simulink model "HevP2ReferenceApplication"  (R2023a)
settings: Solver=ode23tb  StartTime=0  StopTime=1000  RelTol=1e-2  EnableMultiTasking=on
undefined symbols (not defined in the file): at, SOCLast, Stuck
libraries: simulink x5, SignalEditorBlockLib x4, autolibshared x2, FIBlockLib x2
(part 2 of 2)

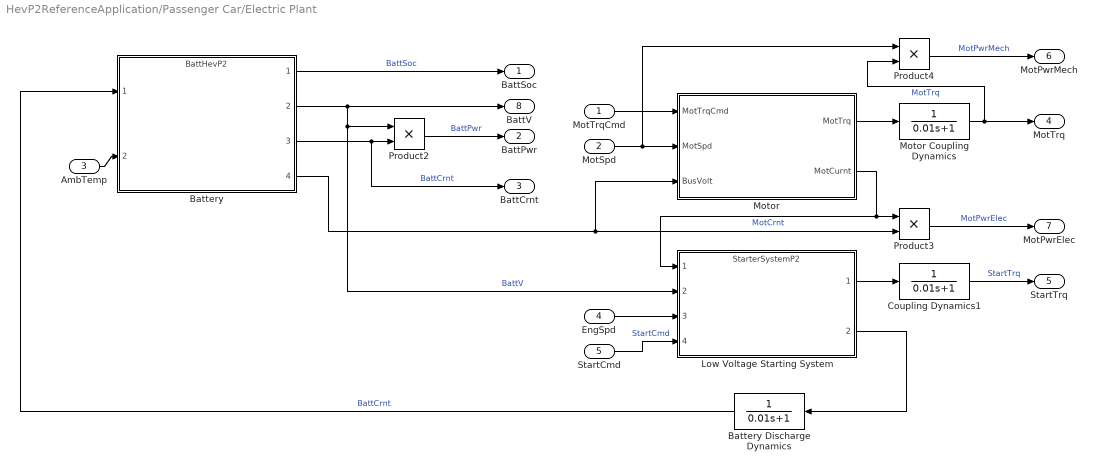
== system HevP2ReferenceApplication/Passenger Car/Electric Plant ==
  MotTrqCmd : Inport
  MotSpd : Inport  Port=2
  AmbTemp : Inport  Port=3
  EngSpd : Inport  Port=4
  StartCmd : Inport  Port=5
  Battery : ModelReference  ModelNameDialog=BattHevP2.slx  SimulationMode=Normal  ModelReferenceVersion=7.0
  Battery Discharge Dynamics : TransferFcn  Denominator=[0.01 1]
  Coupling Dynamics1 : TransferFcn  Denominator=[0.01 1]
  Low Voltage Starting System : ModelReference  ModelNameDialog=StarterSystemP2.slx  SimulationMode=Normal  ModelReferenceVersion=9.1
  Motor : Subsystem  Variant=on  VariantControlMode=label  LabelModeActiveChoice=MotMapped
  Motor Coupling Dynamics : TransferFcn  Denominator=[0.01 1]
  Product2 : Product
  Product3 : Product
  Product4 : Product
  BattSoc : Outport  VectorParamsAs1DForOutWhenUnconnected=off
  BattPwr : Outport  Port=2  VectorParamsAs1DForOutWhenUnconnected=off
  BattCrnt : Outport  Port=3  VectorParamsAs1DForOutWhenUnconnected=off
  MotTrq : Outport  Port=4  VectorParamsAs1DForOutWhenUnconnected=off
  StartTrq : Outport  Port=5  VectorParamsAs1DForOutWhenUnconnected=off
  MotPwrMech : Outport  Port=6  VectorParamsAs1DForOutWhenUnconnected=off
  MotPwrElec : Outport  Port=7  VectorParamsAs1DForOutWhenUnconnected=off
  BattV : Outport  Port=8  VectorParamsAs1DForOutWhenUnconnected=off
  wires:
  Battery/2 -> Low Voltage Starting System/2, Product2/1, BattV/1  "BattV"
  Battery/1 -> BattSoc/1  "BattSoc"
  MotSpd/1 -> Product4/1, Motor/2(MotSpd)
  MotTrqCmd/1 -> Motor/1(MotTrqCmd)
  AmbTemp/1 -> Battery/2
  Product2/1 -> BattPwr/1  "BattPwr"
  Motor/1(MotTrq) -> Motor Coupling Dynamics/1
  Motor Coupling Dynamics/1 -> Product4/2, MotTrq/1  "MotTrq"
  Low Voltage Starting System/2 -> Battery Discharge Dynamics/1
  Motor/2(MotCurnt) -> Low Voltage Starting System/1, Product3/1  "MotCrnt"
  EngSpd/1 -> Low Voltage Starting System/3
  StartCmd/1 -> Low Voltage Starting System/4  "StartCmd"
  Low Voltage Starting System/1 -> Coupling Dynamics1/1
  Product4/1 -> MotPwrMech/1  "MotPwrMech"
  Product3/1 -> MotPwrElec/1  "MotPwrElec"
  Battery Discharge Dynamics/1 -> Battery/1  "BattCrnt"
  Coupling Dynamics1/1 -> StartTrq/1  "StartTrq"
  Battery/3 -> Product2/2, BattCrnt/1  "BattCrnt"
  Battery/4 -> Motor/3(BusVolt), Product3/2

== system HevP2ReferenceApplication/Passenger Car/Electric Plant Input ==
  Ctrl : Inport
  Veh : Inport  Port=2
  Env : Inport  Port=3
  EngFdbk : Inport  Port=4
  Bus Selector : BusSelector  OutputSignals=PtCtrl.MotTrqCmd,PtCtrl.StartCmd
  Bus Selector1 : BusSelector  OutputSignals=MotSpd
  Bus Selector2 : BusSelector  OutputSignals=Temp
  Bus Selector3 : BusSelector  OutputSignals=EngSpd
  First Order Hold : FirstOrderHold  OutputAlgorithm=Fast (Minimize Error)  ErrorTolerance=10e6
  First Order Hold1 : FirstOrderHold  ErrorTolerance=10e6
  MotTrqCmd : Outport  VectorParamsAs1DForOutWhenUnconnected=off
  MotSpd : Outport  Port=2  VectorParamsAs1DForOutWhenUnconnected=off
  AmbTemp : Outport  Port=3  VectorParamsAs1DForOutWhenUnconnected=off
  EngSpd : Outport  Port=4  VectorParamsAs1DForOutWhenUnconnected=off
  StartCmd : Outport  Port=5  VectorParamsAs1DForOutWhenUnconnected=off
  wires:
  First Order Hold1/1 -> StartCmd/1  "StartCmd"
  Bus Selector3/1 -> EngSpd/1  "<EngSpd>"
  EngFdbk/1 -> Bus Selector3/1
  Bus Selector2/1 -> AmbTemp/1  "<Temp>"
  Env/1 -> Bus Selector2/1
  Bus Selector1/1 -> MotSpd/1  "<MotSpd>"
  Veh/1 -> Bus Selector1/1
  Bus Selector/1 -> First Order Hold/1  "<MotTrqCmd>"
  Ctrl/1 -> Bus Selector/1
  First Order Hold/1 -> MotTrqCmd/1  "MotTrqCmd"
  Bus Selector/2 -> First Order Hold1/1  "<StartCmd>"

== system HevP2ReferenceApplication/Passenger Car/Electric Plant Output ==
  BattSoc : Inport
  BattPwr : Inport  Port=2
  BattCrnt : Inport  Port=3
  MotTrq : Inport  Port=4
  StartTrq : Inport  Port=5
  MotPwrMech : Inport  Port=6
  MotPwrElec : Inport  Port=7
  BattV : Inport  Port=8
  Bus Creator1 : BusCreator  Inputs=8
  ElecFdbk : Outport  VectorParamsAs1DForOutWhenUnconnected=off
  wires:
  BattV/1 -> Bus Creator1/8
  MotPwrElec/1 -> Bus Creator1/7
  MotPwrMech/1 -> Bus Creator1/6
  StartTrq/1 -> Bus Creator1/5
  MotTrq/1 -> Bus Creator1/4
  BattCrnt/1 -> Bus Creator1/3
  BattSoc/1 -> Bus Creator1/1
  BattPwr/1 -> Bus Creator1/2
  Bus Creator1/1 -> ElecFdbk/1  "ElecFdbk"

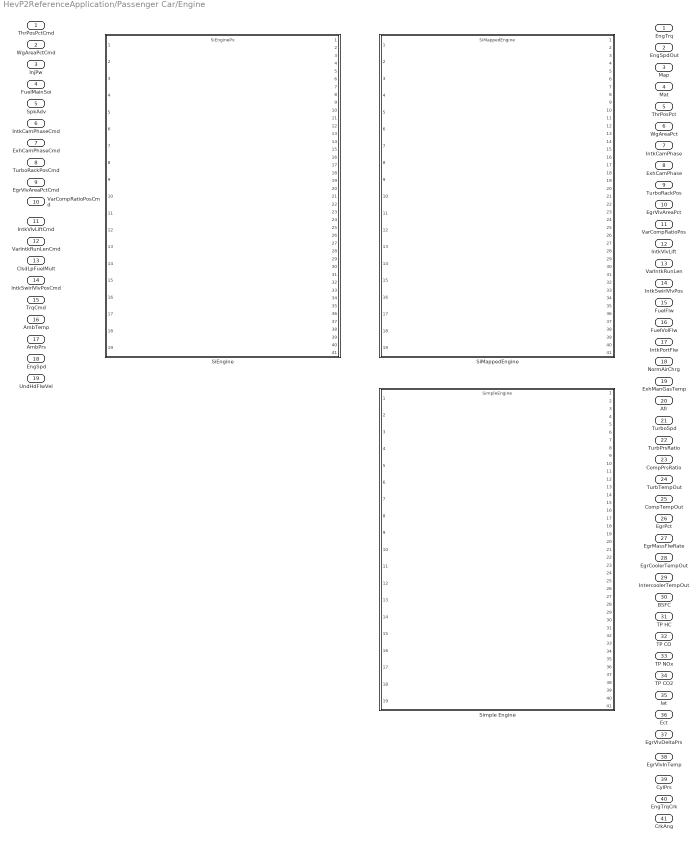
== system HevP2ReferenceApplication/Passenger Car/Engine ==
  ThrPosPctCmd : Inport
  WgAreaPctCmd : Inport  Port=2
  InjPw : Inport  Port=3
  FuelMainSoi : Inport  Port=4
  SpkAdv : Inport  Port=5
  IntkCamPhaseCmd : Inport  Port=6
  ExhCamPhaseCmd : Inport  Port=7
  TurboRackPosCmd : Inport  Port=8
  EgrVlvAreaPctCmd : Inport  Port=9
  VarCompRatioPosCmd : Inport  Port=10
  IntkVlvLiftCmd : Inport  Port=11
  VarIntkRunLenCmd : Inport  Port=12
  ClsdLpFuelMult : Inport  Port=13
  IntkSwirlVlvPosCmd : Inport  Port=14
  TrqCmd : Inport  Port=15
  AmbTemp : Inport  Port=16
  AmbPrs : Inport  Port=17
  EngSpd : Inport  Port=18
  UndHdFlwVel : Inport  Port=19
  SiEngine : ModelReference  ModelNameDialog=SiEnginePx.slx  SimulationMode=Normal  VariantControl=SiEngine  ModelReferenceVersion=6.0
  SiMappedEngine : ModelReference  ModelNameDialog=SiMappedEngine.slx  SimulationMode=Normal  VariantControl=SiMappedEngine  ModelReferenceVersion=6.0
  Simple Engine : ModelReference  ModelNameDialog=SimpleEngine.slx  SimulationMode=Normal  VariantControl=Simple Engine  ModelReferenceVersion=6.0
  EngTrq : Outport  VectorParamsAs1DForOutWhenUnconnected=off
  EngSpdOut : Outport  Port=2  VectorParamsAs1DForOutWhenUnconnected=off
  Map : Outport  Port=3  VectorParamsAs1DForOutWhenUnconnected=off
  Mat : Outport  Port=4  VectorParamsAs1DForOutWhenUnconnected=off
  ThrPosPct : Outport  Port=5  VectorParamsAs1DForOutWhenUnconnected=off
  WgAreaPct : Outport  Port=6  VectorParamsAs1DForOutWhenUnconnected=off
  IntkCamPhase : Outport  Port=7  VectorParamsAs1DForOutWhenUnconnected=off
  ExhCamPhase : Outport  Port=8  VectorParamsAs1DForOutWhenUnconnected=off
  TurboRackPos : Outport  Port=9  VectorParamsAs1DForOutWhenUnconnected=off
  EgrVlvAreaPct : Outport  Port=10  VectorParamsAs1DForOutWhenUnconnected=off
  VarCompRatioPos : Outport  Port=11  VectorParamsAs1DForOutWhenUnconnected=off
  IntkVlvLift : Outport  Port=12  VectorParamsAs1DForOutWhenUnconnected=off
  VarIntkRunLen : Outport  Port=13  VectorParamsAs1DForOutWhenUnconnected=off
  IntkSwirlVlvPos : Outport  Port=14  VectorParamsAs1DForOutWhenUnconnected=off
  FuelFlw : Outport  Port=15  VectorParamsAs1DForOutWhenUnconnected=off
  FuelVolFlw : Outport  Port=16  VectorParamsAs1DForOutWhenUnconnected=off
  IntkPortFlw : Outport  Port=17  VectorParamsAs1DForOutWhenUnconnected=off
  NormAirChrg : Outport  Port=18  VectorParamsAs1DForOutWhenUnconnected=off
  ExhManGasTemp : Outport  Port=19  VectorParamsAs1DForOutWhenUnconnected=off
  Afr : Outport  Port=20  VectorParamsAs1DForOutWhenUnconnected=off
  TurboSpd : Outport  Port=21  VectorParamsAs1DForOutWhenUnconnected=off
  TurbPrsRatio : Outport  Port=22  VectorParamsAs1DForOutWhenUnconnected=off
  CompPrsRatio : Outport  Port=23  VectorParamsAs1DForOutWhenUnconnected=off
  TurbTempOut : Outport  Port=24  VectorParamsAs1DForOutWhenUnconnected=off
  CompTempOut : Outport  Port=25  VectorParamsAs1DForOutWhenUnconnected=off
  EgrPct : Outport  Port=26  VectorParamsAs1DForOutWhenUnconnected=off
  EgrMassFlwRate : Outport  Port=27  VectorParamsAs1DForOutWhenUnconnected=off
  EgrCoolerTempOut : Outport  Port=28  VectorParamsAs1DForOutWhenUnconnected=off
  IntercoolerTempOut : Outport  Port=29  VectorParamsAs1DForOutWhenUnconnected=off
  BSFC : Outport  Port=30  VectorParamsAs1DForOutWhenUnconnected=off
  TP HC : Outport  Port=31  VectorParamsAs1DForOutWhenUnconnected=off
  TP CO : Outport  Port=32  VectorParamsAs1DForOutWhenUnconnected=off
  TP NOx : Outport  Port=33  VectorParamsAs1DForOutWhenUnconnected=off
  TP CO2 : Outport  Port=34  VectorParamsAs1DForOutWhenUnconnected=off
  Iat : Outport  Port=35  VectorParamsAs1DForOutWhenUnconnected=off
  Ect : Outport  Port=36  VectorParamsAs1DForOutWhenUnconnected=off
  EgrVlvDeltaPrs : Outport  Port=37  VectorParamsAs1DForOutWhenUnconnected=off
  EgrVlvInTemp : Outport  Port=38  VectorParamsAs1DForOutWhenUnconnected=off
  CylPrs : Outport  Port=39  VectorParamsAs1DForOutWhenUnconnected=off
  EngTrqCrk : Outport  Port=40  VectorParamsAs1DForOutWhenUnconnected=off
  CrkAng : Outport  Port=41  VectorParamsAs1DForOutWhenUnconnected=off

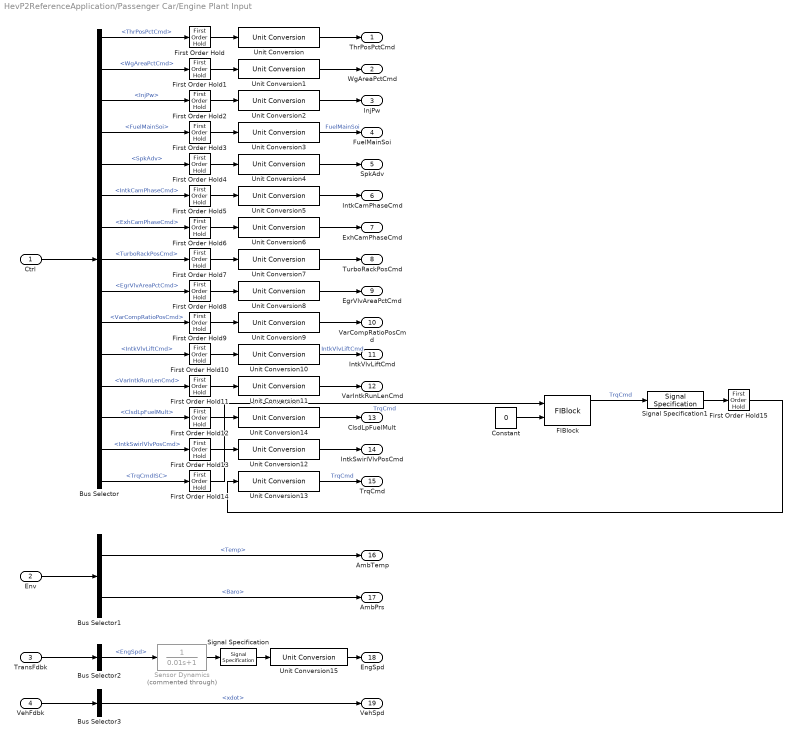
== system HevP2ReferenceApplication/Passenger Car/Engine Plant Input ==
  Ctrl : Inport
  Env : Inport  Port=2
  TransFdbk : Inport  Port=3
  VehFdbk : Inport  Port=4
  Bus Selector : BusSelector  OutputSignals=EngCtrl.ThrPosPctCmd,EngCtrl.WgAreaPctCmd,EngCtrl.InjPw,EngCtrl.FuelMainSoi,EngCtrl.SpkAdv,EngCtrl.IntkCamPhaseCmd,EngCtrl.ExhCamPhaseCmd,EngCtrl.TurboRackPosCmd,EngCtrl.EgrVlvAreaPctCmd,EngCtrl.VarCompRatioPosCmd,EngCtrl.IntkVlvLiftCmd,EngCtrl.VarIntkRunLenCmd,EngCtrl.ClsdLpFuelMult,EngCtrl.IntkSwirlVlvPosCmd,EngCtrl.TrqCmdISC
  Bus Selector1 : BusSelector  OutputSignals=Temp,Baro
  Bus Selector2 : BusSelector  OutputSignals=EngSpd
  Bus Selector3 : BusSelector  OutputSignals=xdot
  Constant : Constant  Value=0
  FIBlock : FIBlockLib/FIBlock  FIBlockName=2  FInjEnable=off  FaultType=Stuck-at  FaultValue=1  FaultEvent=Deterministic  EventValue=50  FaultEffect=Infinite time  EffectValue=0
      settings: SourceProductName=Fault Injection block
  First Order Hold : FirstOrderHold  ErrorTolerance=10e6
  First Order Hold1 : FirstOrderHold  ErrorTolerance=10e6
  First Order Hold{3..14} (12 alike) : FirstOrderHold  ErrorTolerance=10e6  AllowContinuousInput=on
  First Order Hold15 : FirstOrderHold  ErrorTolerance=inf
  First Order Hold2 : FirstOrderHold  ErrorTolerance=10e6
  Sensor Dynamics : TransferFcn  Commented=through  Denominator=[0.01 1]
  Signal Specification : SignalSpecification  Unit=rad/s
  Signal Specification1 : SignalSpecification  Unit=N*m
  Unit Conversion{,1..12,14..15} (15 alike) : UnitConversion
  Unit Conversion13 : UnitConversion  OutputType=Inherit: Inherit via back propagation
  ThrPosPctCmd : Outport  VectorParamsAs1DForOutWhenUnconnected=off
  WgAreaPctCmd : Outport  Port=2  VectorParamsAs1DForOutWhenUnconnected=off
  InjPw : Outport  Port=3  VectorParamsAs1DForOutWhenUnconnected=off
  FuelMainSoi : Outport  Port=4  VectorParamsAs1DForOutWhenUnconnected=off
  SpkAdv : Outport  Port=5  VectorParamsAs1DForOutWhenUnconnected=off
  IntkCamPhaseCmd : Outport  Port=6  VectorParamsAs1DForOutWhenUnconnected=off
  ExhCamPhaseCmd : Outport  Port=7  VectorParamsAs1DForOutWhenUnconnected=off
  TurboRackPosCmd : Outport  Port=8  VectorParamsAs1DForOutWhenUnconnected=off
  EgrVlvAreaPctCmd : Outport  Port=9  VectorParamsAs1DForOutWhenUnconnected=off
  VarCompRatioPosCmd : Outport  Port=10  VectorParamsAs1DForOutWhenUnconnected=off
  IntkVlvLiftCmd : Outport  Port=11  VectorParamsAs1DForOutWhenUnconnected=off
  VarIntkRunLenCmd : Outport  Port=12  VectorParamsAs1DForOutWhenUnconnected=off
  ClsdLpFuelMult : Outport  Port=13  VectorParamsAs1DForOutWhenUnconnected=off
  IntkSwirlVlvPosCmd : Outport  Port=14  VectorParamsAs1DForOutWhenUnconnected=off
  TrqCmd : Outport  Port=15  VectorParamsAs1DForOutWhenUnconnected=off
  AmbTemp : Outport  Port=16  VectorParamsAs1DForOutWhenUnconnected=off
  AmbPrs : Outport  Port=17  VectorParamsAs1DForOutWhenUnconnected=off
  EngSpd : Outport  Port=18  VectorParamsAs1DForOutWhenUnconnected=off
  VehSpd : Outport  Port=19  VectorParamsAs1DForOutWhenUnconnected=off
  wires:
  Env/1 -> Bus Selector1/1
  Bus Selector1/2 -> AmbPrs/1  "<Baro>"
  TransFdbk/1 -> Bus Selector2/1
  Bus Selector2/1 -> Sensor Dynamics/1  "<EngSpd>"
  Bus Selector1/1 -> AmbTemp/1  "<Temp>"
  VehFdbk/1 -> Bus Selector3/1
  Bus Selector3/1 -> VehSpd/1  "<xdot>"
  Sensor Dynamics/1 -> Signal Specification/1
  Ctrl/1 -> Bus Selector/1
  First Order Hold13/1 -> Unit Conversion12/1
  First Order Hold12/1 -> Unit Conversion14/1
  First Order Hold11/1 -> Unit Conversion11/1
  First Order Hold10/1 -> Unit Conversion10/1
  First Order Hold9/1 -> Unit Conversion9/1
  First Order Hold3/1 -> Unit Conversion3/1
  First Order Hold/1 -> Unit Conversion/1
  First Order Hold1/1 -> Unit Conversion1/1
  First Order Hold2/1 -> Unit Conversion2/1
  First Order Hold4/1 -> Unit Conversion4/1
  First Order Hold5/1 -> Unit Conversion5/1
  First Order Hold6/1 -> Unit Conversion6/1
  First Order Hold7/1 -> Unit Conversion7/1
  First Order Hold8/1 -> Unit Conversion8/1
  Bus Selector/1 -> First Order Hold/1  "<ThrPosPctCmd>"
  Bus Selector/2 -> First Order Hold1/1  "<WgAreaPctCmd>"
  Bus Selector/3 -> First Order Hold2/1  "<InjPw>"
  Bus Selector/4 -> First Order Hold3/1  "<FuelMainSoi>"
  Bus Selector/5 -> First Order Hold4/1  "<SpkAdv>"
  Bus Selector/6 -> First Order Hold5/1  "<IntkCamPhaseCmd>"
  Bus Selector/7 -> First Order Hold6/1  "<ExhCamPhaseCmd>"
  Bus Selector/8 -> First Order Hold7/1  "<TurboRackPosCmd>"
  Bus Selector/9 -> First Order Hold8/1  "<EgrVlvAreaPctCmd>"
  Bus Selector/10 -> First Order Hold9/1  "<VarCompRatioPosCmd>"
  Bus Selector/11 -> First Order Hold10/1  "<IntkVlvLiftCmd>"
  Bus Selector/12 -> First Order Hold11/1  "<VarIntkRunLenCmd>"
  Bus Selector/13 -> First Order Hold12/1  "<ClsdLpFuelMult>"
  Bus Selector/14 -> First Order Hold13/1  "<IntkSwirlVlvPosCmd>"
  Bus Selector/15 -> First Order Hold14/1  "<TrqCmdISC>"
  Unit Conversion11/1 -> VarIntkRunLenCmd/1
  Unit Conversion8/1 -> EgrVlvAreaPctCmd/1
  Unit Conversion12/1 -> IntkSwirlVlvPosCmd/1
  Unit Conversion14/1 -> ClsdLpFuelMult/1
  Unit Conversion/1 -> ThrPosPctCmd/1
  Unit Conversion1/1 -> WgAreaPctCmd/1
  Unit Conversion3/1 -> FuelMainSoi/1  "FuelMainSoi"
  Unit Conversion2/1 -> InjPw/1
  Unit Conversion9/1 -> VarCompRatioPosCmd/1
  Unit Conversion4/1 -> SpkAdv/1
  Unit Conversion7/1 -> TurboRackPosCmd/1
  Unit Conversion13/1 -> TrqCmd/1  "TrqCmd"
  Unit Conversion10/1 -> IntkVlvLiftCmd/1  "IntkVlvLiftCmd"
  Unit Conversion6/1 -> ExhCamPhaseCmd/1
  Unit Conversion5/1 -> IntkCamPhaseCmd/1
  Unit Conversion15/1 -> EngSpd/1
  Signal Specification/1 -> Unit Conversion15/1
  First Order Hold14/1 -> FIBlock/1  "TrqCmd"
  FIBlock/1 -> Signal Specification1/1  "TrqCmd"
  Constant/1 -> FIBlock/2
  Signal Specification1/1 -> First Order Hold15/1
  First Order Hold15/1 -> Unit Conversion13/1

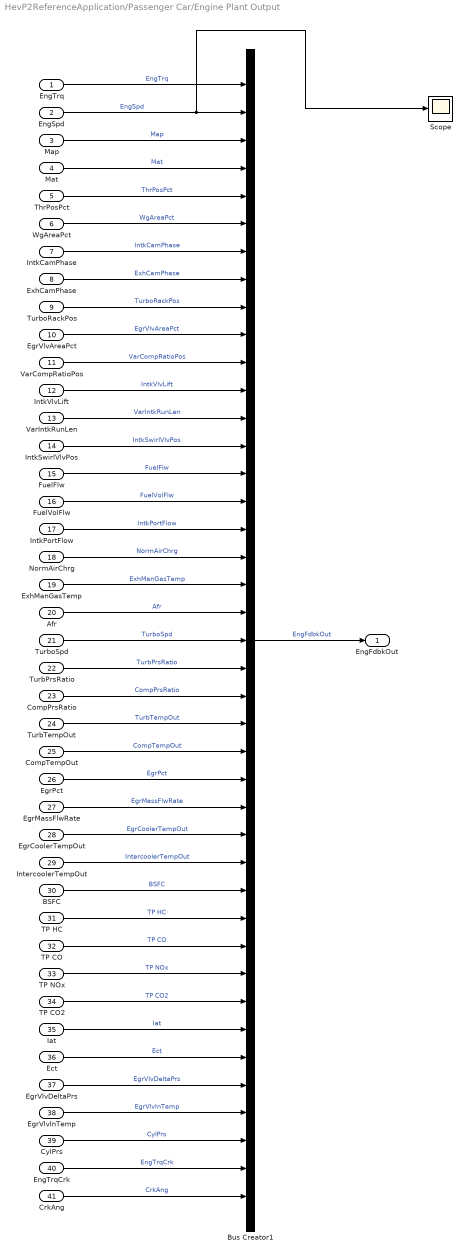
== system HevP2ReferenceApplication/Passenger Car/Engine Plant Output ==
  EngTrq : Inport
  EngSpd : Inport  Port=2
  Map : Inport  Port=3
  Mat : Inport  Port=4
  ThrPosPct : Inport  Port=5
  WgAreaPct : Inport  Port=6
  IntkCamPhase : Inport  Port=7
  ExhCamPhase : Inport  Port=8
  TurboRackPos : Inport  Port=9
  EgrVlvAreaPct : Inport  Port=10
  VarCompRatioPos : Inport  Port=11
  IntkVlvLift : Inport  Port=12
  VarIntkRunLen : Inport  Port=13
  IntkSwirlVlvPos : Inport  Port=14
  FuelFlw : Inport  Port=15
  FuelVolFlw : Inport  Port=16
  IntkPortFlow : Inport  Port=17
  NormAirChrg : Inport  Port=18
  ExhManGasTemp : Inport  Port=19
  Afr : Inport  Port=20
  TurboSpd : Inport  Port=21
  TurbPrsRatio : Inport  Port=22
  CompPrsRatio : Inport  Port=23
  TurbTempOut : Inport  Port=24
  CompTempOut : Inport  Port=25
  EgrPct : Inport  Port=26
  EgrMassFlwRate : Inport  Port=27
  EgrCoolerTempOut : Inport  Port=28
  IntercoolerTempOut : Inport  Port=29
  BSFC : Inport  Port=30
  TP HC : Inport  Port=31
  TP CO : Inport  Port=32
  TP NOx : Inport  Port=33
  TP CO2 : Inport  Port=34
  Iat : Inport  Port=35
  Ect : Inport  Port=36
  EgrVlvDeltaPrs : Inport  Port=37
  EgrVlvInTemp : Inport  Port=38
  CylPrs : Inport  Port=39
  EngTrqCrk : Inport  Port=40
  CrkAng : Inport  Port=41
  Bus Creator1 : BusCreator  Inputs=41
  Scope : Scope
  EngFdbkOut : Outport  VectorParamsAs1DForOutWhenUnconnected=off
  wires:
  CrkAng/1 -> Bus Creator1/41  "CrkAng"
  EngTrqCrk/1 -> Bus Creator1/40  "EngTrqCrk"
  CylPrs/1 -> Bus Creator1/39  "CylPrs"
  EgrVlvInTemp/1 -> Bus Creator1/38  "EgrVlvInTemp"
  EgrVlvDeltaPrs/1 -> Bus Creator1/37  "EgrVlvDeltaPrs"
  Ect/1 -> Bus Creator1/36  "Ect"
  Iat/1 -> Bus Creator1/35  "Iat"
  TP CO2/1 -> Bus Creator1/34  "TP CO2"
  TP NOx/1 -> Bus Creator1/33  "TP NOx"
  TP CO/1 -> Bus Creator1/32  "TP CO"
  TP HC/1 -> Bus Creator1/31  "TP HC"
  BSFC/1 -> Bus Creator1/30  "BSFC"
  IntercoolerTempOut/1 -> Bus Creator1/29  "IntercoolerTempOut"
  EgrCoolerTempOut/1 -> Bus Creator1/28  "EgrCoolerTempOut"
  EgrMassFlwRate/1 -> Bus Creator1/27  "EgrMassFlwRate"
  EgrPct/1 -> Bus Creator1/26  "EgrPct"
  CompTempOut/1 -> Bus Creator1/25  "CompTempOut"
  TurbTempOut/1 -> Bus Creator1/24  "TurbTempOut"
  CompPrsRatio/1 -> Bus Creator1/23  "CompPrsRatio"
  TurbPrsRatio/1 -> Bus Creator1/22  "TurbPrsRatio"
  TurboSpd/1 -> Bus Creator1/21  "TurboSpd"
  Afr/1 -> Bus Creator1/20  "Afr"
  ExhManGasTemp/1 -> Bus Creator1/19  "ExhManGasTemp"
  NormAirChrg/1 -> Bus Creator1/18  "NormAirChrg"
  IntkPortFlow/1 -> Bus Creator1/17  "IntkPortFlow"
  FuelVolFlw/1 -> Bus Creator1/16  "FuelVolFlw"
  FuelFlw/1 -> Bus Creator1/15  "FuelFlw"
  IntkSwirlVlvPos/1 -> Bus Creator1/14  "IntkSwirlVlvPos"
  Bus Creator1/1 -> EngFdbkOut/1  "EngFdbkOut"
  EgrVlvAreaPct/1 -> Bus Creator1/10  "EgrVlvAreaPct"
  ExhCamPhase/1 -> Bus Creator1/8  "ExhCamPhase"
  IntkCamPhase/1 -> Bus Creator1/7  "IntkCamPhase"
  EngSpd/1 -> Scope/1, Bus Creator1/2  "EngSpd"
  Map/1 -> Bus Creator1/3  "Map"
  Mat/1 -> Bus Creator1/4  "Mat"
  EngTrq/1 -> Bus Creator1/1  "EngTrq"
  ThrPosPct/1 -> Bus Creator1/5  "ThrPosPct"
  TurboRackPos/1 -> Bus Creator1/9  "TurboRackPos"
  WgAreaPct/1 -> Bus Creator1/6  "WgAreaPct"
  VarCompRatioPos/1 -> Bus Creator1/11  "VarCompRatioPos"
  IntkVlvLift/1 -> Bus Creator1/12  "IntkVlvLift"
  VarIntkRunLen/1 -> Bus Creator1/13  "VarIntkRunLen"

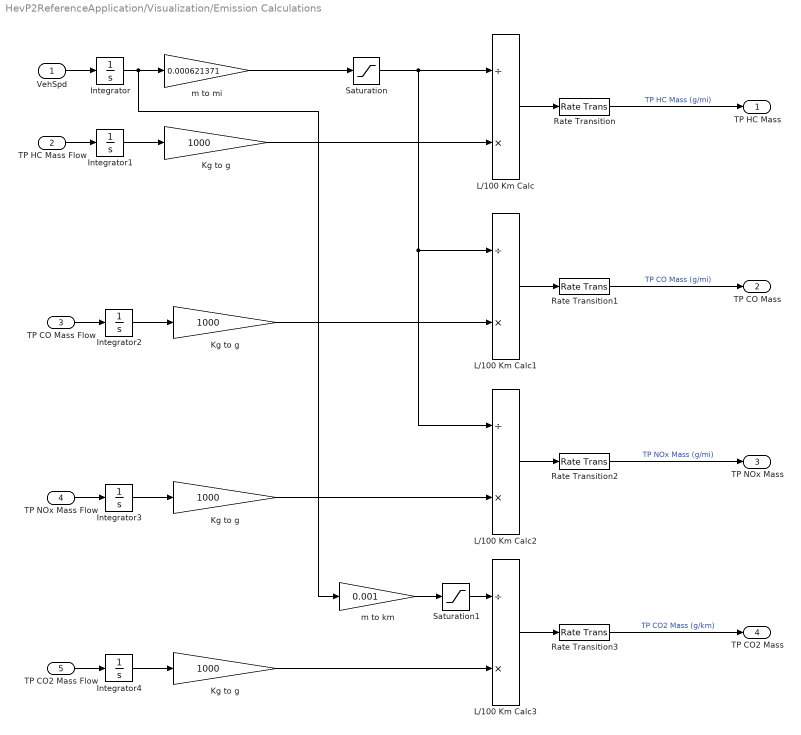
== system HevP2ReferenceApplication/Visualization/Emission Calculations ==
  VehSpd : Inport
  TP HC Mass Flow : Inport  Port=2
  TP CO Mass Flow : Inport  Port=3
  TP NOx Mass Flow : Inport  Port=4
  TP CO2 Mass Flow : Inport  Port=5
  Integrator{,1..4} (5 alike) : Integrator
  Kg to g : Gain  Gain=1000
  "Kg to g " : Gain  Gain=1000
  "Kg to g  " : Gain  Gain=1000
  "Kg to g   " : Gain  Gain=1000
  L/100 Km Calc{,1..3} (4 alike) : Product  Inputs=/*
  Rate Transition{,1..3} (4 alike) : RateTransition  Deterministic=off
  Saturation : Saturate  UpperLimit=Inf  LowerLimit=0.2
  Saturation1 : Saturate  UpperLimit=Inf  LowerLimit=1
  m to km : Gain  Gain=0.001
  m to mi : Gain  Gain=0.000621371
  TP HC Mass : Outport  VectorParamsAs1DForOutWhenUnconnected=off
  TP CO Mass : Outport  Port=2  VectorParamsAs1DForOutWhenUnconnected=off
  TP NOx Mass : Outport  Port=3  VectorParamsAs1DForOutWhenUnconnected=off
  TP CO2 Mass : Outport  Port=4  VectorParamsAs1DForOutWhenUnconnected=off
  wires:
  L/100 Km Calc/1 -> Rate Transition/1
  VehSpd/1 -> Integrator/1
  m to mi/1 -> Saturation/1
  Saturation/1 -> L/100 Km Calc2/1, L/100 Km Calc1/1, L/100 Km Calc/1
  TP HC Mass Flow/1 -> Integrator1/1
  Integrator1/1 -> Kg to g/1
  Integrator/1 -> m to km/1, m to mi/1
  Kg to g/1 -> L/100 Km Calc/2
  TP CO Mass Flow/1 -> Integrator2/1
  Integrator2/1 -> "Kg to g "/1
  "Kg to g "/1 -> L/100 Km Calc1/2
  TP NOx Mass Flow/1 -> Integrator3/1
  Integrator3/1 -> "Kg to g  "/1
  "Kg to g  "/1 -> L/100 Km Calc2/2
  L/100 Km Calc1/1 -> Rate Transition1/1
  L/100 Km Calc2/1 -> Rate Transition2/1
  TP CO2 Mass Flow/1 -> Integrator4/1
  Integrator4/1 -> "Kg to g   "/1
  "Kg to g   "/1 -> L/100 Km Calc3/2
  L/100 Km Calc3/1 -> Rate Transition3/1
  Saturation1/1 -> L/100 Km Calc3/1
  m to km/1 -> Saturation1/1
  Rate Transition/1 -> TP HC Mass/1  "TP HC Mass (g/mi)"
  Rate Transition1/1 -> TP CO Mass/1  "TP CO Mass (g/mi)"
  Rate Transition2/1 -> TP NOx Mass/1  "TP NOx Mass (g/mi)"
  Rate Transition3/1 -> TP CO2 Mass/1  "TP CO2 Mass (g/km)"

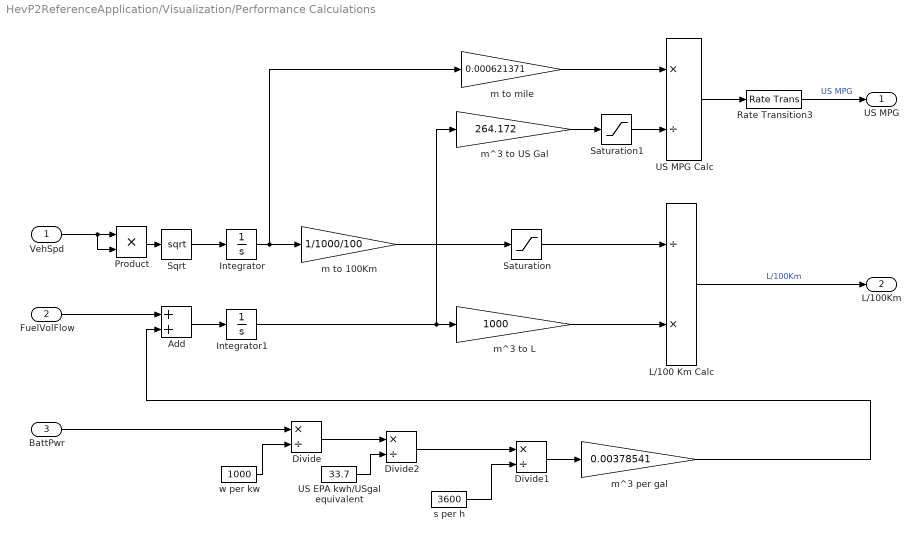
== system HevP2ReferenceApplication/Visualization/Performance Calculations ==
  VehSpd : Inport
  FuelVolFlow : Inport  Port=2
  BattPwr : Inport  Port=3
  Add : Sum
  Divide : Product  Inputs=*/
  Divide1 : Product  Inputs=*/
  Divide2 : Product  Inputs=*/
  Integrator : Integrator
  Integrator1 : Integrator
  L/100 Km Calc : Product  Inputs=/*
  Product : Product
  Rate Transition3 : RateTransition  Deterministic=off
  Saturation : Saturate  UpperLimit=Inf  LowerLimit=0.001
  Saturation1 : Saturate  UpperLimit=Inf  LowerLimit=1e-3
  Sqrt : Sqrt
  US EPA kwh/USgal equivalent : Constant  Value=33.7
  US MPG Calc : Product  Inputs=*/
  m to 100Km : Gain  Gain=1/1000/100
  m to mile : Gain  Gain=0.000621371
  m^3 per gal : Gain  Gain=0.00378541
  m^3 to L : Gain  Gain=1000
  m^3 to US Gal : Gain  Gain=264.172
  s per h : Constant  Value=3600
  w per kw : Constant  Value=1000
  US MPG : Outport  VectorParamsAs1DForOutWhenUnconnected=off
  L/100Km : Outport  Port=2  VectorParamsAs1DForOutWhenUnconnected=off
  wires:
  m^3 to US Gal/1 -> Saturation1/1
  m^3 to L/1 -> L/100 Km Calc/2
  Integrator/1 -> m to mile/1, m to 100Km/1
  m to mile/1 -> US MPG Calc/1
  FuelVolFlow/1 -> Add/1
  Integrator1/1 -> m^3 to US Gal/1, m^3 to L/1
  Saturation/1 -> L/100 Km Calc/1
  m to 100Km/1 -> Saturation/1
  L/100 Km Calc/1 -> L/100Km/1  "L/100Km"
  US MPG Calc/1 -> Rate Transition3/1
  Saturation1/1 -> US MPG Calc/2
  Rate Transition3/1 -> US MPG/1  "US MPG"
  w per kw/1 -> Divide/2
  Divide/1 -> Divide2/1
  Divide2/1 -> Divide1/1
  s per h/1 -> Divide1/2
  Divide1/1 -> m^3 per gal/1
  Add/1 -> Integrator1/1
  m^3 per gal/1 -> Add/2
  US EPA kwh/USgal equivalent/1 -> Divide2/2
  BattPwr/1 -> Divide/1
  Sqrt/1 -> Integrator/1
  Product/1 -> Sqrt/1
  VehSpd/1 -> Product/2, Product/1

== system HevP2ReferenceApplication/Controllers/PCM Input/Ending SOC Tuning ==
  BattSOC : Inport
  Ending SOC Tuning Active : Subsystem  InitFcn=|  VariantControl=1  mask{SOCTarget=60}
      | if ~exist('SOCLast','var')
      |    assignin('base','SOCLast',str2num(get_param(gcb,'SOCTarget')));
      | end
  Ending SOC Tuning Inactive : Subsystem  VariantControl=0
  BattSOCTune : Outport

== system HevP2ReferenceApplication/Controllers/Powertrain Control Module (PCM)/Hybrid Control Module (HCM) ==
  AccelPdl : Inport
  DecelPdl : Inport  Port=2
  VehSpdFdbk : Inport  Port=3
  EngSpdFdbk : Inport  Port=4
  BattSoc : Inport  Port=5
  BattPwr : Inport  Port=6
  MtrSpd : Inport  Port=7
  EngTrqOut : Inport  Port=8
  Cltch1State : Inport  Port=9
  Cltch2State : Inport  Port=10
  Chrg : Inport  Port=11
  BattVolt : Inport  Port=12
  TransGear : Inport  Port=13
  Optimal Control : ModelReference  ModelNameDialog=HevP2OptimalController.slx  SimulationMode=Normal  VariantControl=OptimalControl  ModelReferenceVersion=6.1
  Rule-Based Control : ModelReference  ModelNameDialog=HevP2PowertrainController.slx  SimulationMode=Normal  VariantControl=RuleBasedControl  ModelReferenceVersion=6.0
  EngTrqCmd : Outport  VectorParamsAs1DForOutWhenUnconnected=off
  MtrTrqCmd : Outport  Port=2  VectorParamsAs1DForOutWhenUnconnected=off
  BrkCmd : Outport  Port=3  VectorParamsAs1DForOutWhenUnconnected=off
  Cltch1Cmd : Outport  Port=4  VectorParamsAs1DForOutWhenUnconnected=off
  StartCmd : Outport  Port=5  VectorParamsAs1DForOutWhenUnconnected=off
  Neutral : Outport  Port=6  VectorParamsAs1DForOutWhenUnconnected=off
  WhlTrqCmd : Outport  Port=7  VectorParamsAs1DForOutWhenUnconnected=off

== system HevP2ReferenceApplication/Longitudinal Driver/Longitudinal Driver/Hill Hold ==
  xdotref : Inport
  VehFdbk : Inport  Port=2
  Grade : Inport  Port=3
  Abs : Abs  ZeroCross=off  SaturateOnIntegerOverflow=off
  Abs1 : Abs  ZeroCross=off  SaturateOnIntegerOverflow=off
  Bus Selector : BusSelector  OutputSignals=Eng.EngFdbk.EngSpd,Elec.BattSoc,Veh.xdot
  Compare To Constant : simulink/Logic and Bit Operations/Compare To Constant  relop=<=  const=.1  OutDataTypeStr=boolean  ZeroCross=off
  Compare To Constant1 : simulink/Logic and Bit Operations/Compare To Constant  relop=>=  const=.1  OutDataTypeStr=boolean  ZeroCross=off
  Compare To Constant2 : simulink/Logic and Bit Operations/Compare To Constant  relop=<=  const=500  OutDataTypeStr=boolean  ZeroCross=off
  Compare To Constant3 : simulink/Logic and Bit Operations/Compare To Constant  relop=<=  const=5  OutDataTypeStr=boolean  ZeroCross=off
  Compare To Constant4 : simulink/Logic and Bit Operations/Compare To Constant  relop=<=  const=.1  OutDataTypeStr=boolean  ZeroCross=off
  Data Type Conversion1 : DataTypeConversion  SaturateOnIntegerOverflow=off  RndMeth=Floor
  Logical Operator : Logic  AllPortsSameDT=off  OutDataTypeStr=boolean
  Logical Operator1 : Logic  Inputs=3  AllPortsSameDT=off  OutDataTypeStr=boolean
  Logical Operator2 : Logic  Operator=OR  AllPortsSameDT=off  OutDataTypeStr=boolean
  EnblDecelOvr : Outport
  DecelOvrCmd : Outport  Port=2
  wires:
  Logical Operator2/1 -> Data Type Conversion1/1, EnblDecelOvr/1
  Data Type Conversion1/1 -> DecelOvrCmd/1
  xdotref/1 -> Abs/1
  Abs/1 -> Compare To Constant/1
  Grade/1 -> Abs1/1
  Compare To Constant/1 -> Logical Operator/1
  Abs1/1 -> Compare To Constant1/1
  Compare To Constant1/1 -> Logical Operator/2
  Compare To Constant2/1 -> Logical Operator1/1
  Compare To Constant3/1 -> Logical Operator1/2
  Logical Operator1/1 -> Logical Operator2/1
  Logical Operator/1 -> Logical Operator2/2
  Compare To Constant4/1 -> Logical Operator1/3
  VehFdbk/1 -> Bus Selector/1
  Bus Selector/1 -> Compare To Constant2/1  "<EngSpd>"
  Bus Selector/2 -> Compare To Constant3/1  "<BattSoc>"
  Bus Selector/3 -> Compare To Constant4/1  "<xdot>"

== system HevP2ReferenceApplication/Longitudinal Driver/Longitudinal Driver/Optional Stationary Charging ==
  note: Setup for FTP75, allow charging
      | between 1490-1860 secs when
      | vehicle is stopped
  Charge Profile : SignalEditorBlockLib/Signal Editor  FileName=ChargeProfile.mat  ActiveScenario=Group_1  ActiveSignal=IGSW  IsBus=off  OutputBusObjectStr=Bus: BusObject  SampleTime=0  OutputAfterFinalValue=Extrapolation  Unit=inherit  PreserveSignalName=on  ApplySigPropsToAllScenarios=on
  Constant1 : Constant  Value=false
  Data Type Conversion1 : DataTypeConversion  OutDataTypeStr=boolean  SaturateOnIntegerOverflow=off  RndMeth=Floor
  Manual Switch1 : ManualSwitch
  Charge : Outport  VectorParamsAs1DForOutWhenUnconnected=off
  wires:
  Constant1/1 -> Manual Switch1/1
  Data Type Conversion1/1 -> Manual Switch1/2
  Charge Profile/1 -> Data Type Conversion1/1
  Manual Switch1/1 -> Charge/1  "Charge"

== system HevP2ReferenceApplication/Longitudinal Driver/Open Loop/Optional Stationary Charging ==
  note: Setup for FTP75, allow charging
      | between 1490-1860 secs when
      | vehicle is stopped
  Charge Profile : SignalEditorBlockLib/Signal Editor  FileName=ChargeProfile.mat  ActiveScenario=Group_1  ActiveSignal=IGSW  IsBus=off  OutputBusObjectStr=Bus: BusObject  SampleTime=0  OutputAfterFinalValue=Extrapolation  Unit=inherit  PreserveSignalName=on  ApplySigPropsToAllScenarios=on
  Constant1 : Constant  Value=false
  Data Type Conversion1 : DataTypeConversion  OutDataTypeStr=boolean  SaturateOnIntegerOverflow=off  RndMeth=Floor
  Manual Switch1 : ManualSwitch
  Charge : Outport  VectorParamsAs1DForOutWhenUnconnected=off
  wires:
  Constant1/1 -> Manual Switch1/1
  Data Type Conversion1/1 -> Manual Switch1/2
  Charge Profile/1 -> Data Type Conversion1/1
  Manual Switch1/1 -> Charge/1  "Charge"

== system HevP2ReferenceApplication/Passenger Car/Electric Plant/Motor ==
  MotTrqCmd : Inport
  MotSpd : Inport  Port=2
  BusVolt : Inport  Port=3
  MotDynamic : ModelReference  ModelNameDialog=MotDynamicP2.slx  SimulationMode=Normal  VariantControl=MotDynamic  ModelReferenceVersion=9.0
  MotMapped : ModelReference  ModelNameDialog=MotMappedP2.slx  SimulationMode=Normal  VariantControl=MotMapped  ModelReferenceVersion=8.0
  MotTrq : Outport  VectorParamsAs1DForOutWhenUnconnected=off
  MotCurnt : Outport  Port=2  VectorParamsAs1DForOutWhenUnconnected=off

== system HevP2ReferenceApplication/Controllers/PCM Input/Ending SOC Tuning/Ending SOC Tuning Active ==
  BattSOC : Inport
  Constant : Constant  Value=SOCLast
  Constant1 : Constant  Value=SOCTarget
  Gain : Gain  Gain=0.5
  Sum : Sum  Inputs=|+-
  Sum1 : Sum  Inputs=|+-
  To Workspace : ToWorkspace  VariableName=SOCLast  SampleTime=-1
      settings: MaxDataPoints=1
  BattSOCTune : Outport
  wires:
  BattSOC/1 -> Sum1/1, To Workspace/1
  Constant1/1 -> Sum/1
  Constant/1 -> Sum/2
  Sum/1 -> Gain/1
  Sum1/1 -> BattSOCTune/1
  Gain/1 -> Sum1/2

== system HevP2ReferenceApplication/Controllers/PCM Input/Ending SOC Tuning/Ending SOC Tuning Inactive ==
  BattSOC : Inport
  BattSOCTune : Outport
  wires:
  BattSOC/1 -> BattSOCTune/1
